simulink model "testF4"  (R2021a)
settings: Solver=FixedStepAuto  StartTime=0.0  StopTime=10.0  RelTol=1e-3  EnableMultiTasking=on
undefined symbols (not defined in the file): ChargingCurrentRequest, DrivingCurrentRqst, OpenCircuitInjection, ShortCircuitInjection, SystemState, SystemState_t
settings Model: Creator=miche  LastModifiedBy=miche
settings OptimizationCC: EnhancedBackFolding=on  PassReuseOutputArgsAs=Individual arguments  ZeroExternalMemoryAtStartup=off  ZeroInternalMemoryAtStartup=off  MaxStackSize=64  OptimizeBlockOrder=speed  DifferentSizesBufferReuse=on  OptimizationCustomize=off  EfficientTunableParamExpr=on
settings DebuggingCC: ParameterTunabilityLossMsg=error  BusObjectLabelMismatch=error
settings HardwareCC: ProdBitPerPointer=32  ProdBitPerSizeT=32  ProdBitPerPtrDiffT=32  ProdLargestAtomicInteger=Long  ProdLargestAtomicFloat=Double  ProdWordSize=32  ProdHWDeviceType=ARM Compatible->ARM Cortex
settings SFSimCC: MATLABDynamicMemAlloc=off
settings RTWCC: SystemTargetFile=ert.tlc  HardwareBoard=STM32F4-Discovery  TemplateMakefile=ert_default_tmf  Toolchain=GNU Tools for ARM Embedded Processors
settings CodeAppCC: ForceParamTrailComments=on  IgnoreCustomStorageClasses=off  OperatorAnnotations=on  SimulinkDataObjDesc=on  SFDataObjDesc=on  InsertBlockDesc=on
settings ERTTargetCC: CodeReplacementLibrary=ARM Cortex-M (Optimized)  ExtModeTransport=1  ExtModeMexFile=ext_serial_win32_comm

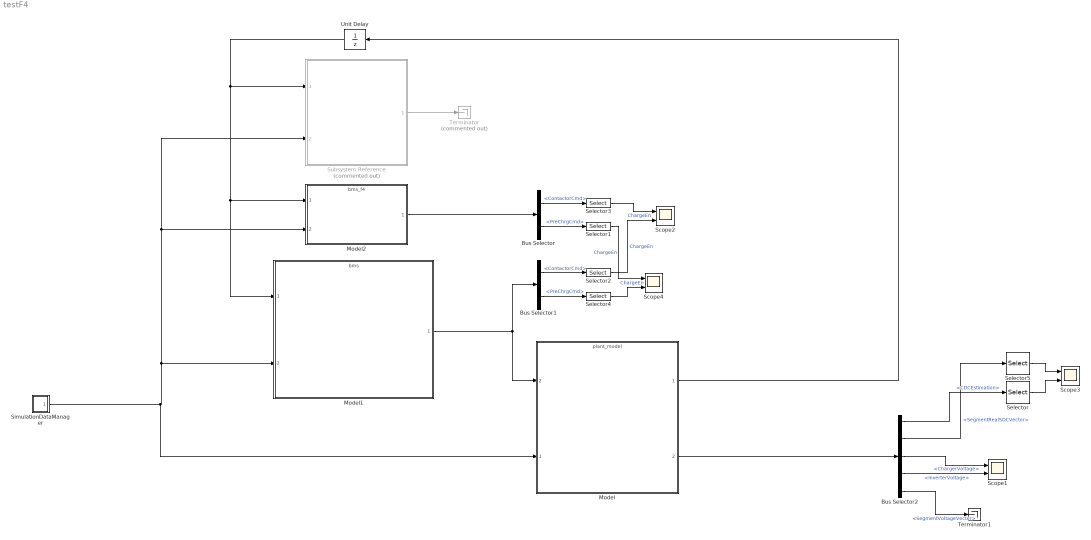
== system testF4 ==
  Bus Selector : BusSelector  OutputSignals=BMSContactorModuleCmd.ContactorCmd,BMSContactorModuleCmd.PreChrgCmd
  Bus Selector1 : BusSelector  OutputSignals=BMSContactorModuleCmd.ContactorCmd,BMSContactorModuleCmd.PreChrgCmd
  Bus Selector2 : BusSelector  OutputSignals=BusSOCEstimation.CDCEstimation,BMSBatteryPackData.SegmentRealSOCVector,SimulationChargerData.ChargerVoltage,SimulationInverterData.InverterVoltage,BMSBatteryPackData.SegmentVoltageVector
  Model : ModelReference  ModelNameDialog=plant_model.slx  SimulationMode=Normal  ModelReferenceVersion=1.26
      settings: PortSchema="{\"entries\":[{\"content\":{\"sides\":[{\"content\":{\"connectorIds\":[\"In2\",\"In1\"]},\"type\":\"ConnectorPlacement.EquallySpacedRectSide\",\"uuid\":\"0f2d7512-e5af-4bec-8093-bd7de674fa12\"},{\"content\":{\"connectorIds\":[\"Out1\",\"Out2\"],\"side\":\"RIGHT\"},\"type\":\"ConnectorPlacement.EquallySpacedRectSide\",\"uuid\":\"ba98a958-4ea7-42df-a4be-bb9f55905ebf\"},{\"content\":{\"connectorIds\":[],\"side\":\"TOP\"},\"type\":\"ConnectorPlacement.EquallySpacedRectSide\",\"uuid\":\"7b43f5d7-e5ff-427f-a248-64d763618be9\"}]},\"type\":\"ConnectorPlacement.EquallySpacedConnector\",\"uuid\":\"924ca3d4-4439-427a-b78a-546ec9901955\"}],\"packageUris\":[\"http://schema.mathworks.com/mf0/Connector/R2020b\"],\"version\":\"1.0\"}"
      mask Display: image('$imagefile'); % Use "Edit Image" on toolstrip to change.
  Model1 : ModelReference  ModelNameDialog=bms.slx  SimulationMode=Normal  ModelReferenceVersion=1.35
      mask Display: image('$imagefile'); % Use "Edit Image" on toolstrip to change.
  Model2 : ModelReference  ModelNameDialog=bms_f4.slx  SimulationMode=Processor-in-the-loop (PIL)  CodeInterface=Top model  ModelReferenceVersion=1.33
  Scope{1..4} (4 alike) : Scope  NumInputPorts=2
  Selector : Selector  NumberOfDimensions=2  InputPortWidth=3  IndexOptions=Index vector (dialog),Index vector (dialog)  Indices=1,1  OutputSizes=1,1
  Selector1 : Selector  InputPortWidth=2  IndexOptions=Index vector (dialog)  Indices=1  OutputSizes=1
  Selector2 : Selector  InputPortWidth=3  IndexOptions=Index vector (dialog)  Indices=1  OutputSizes=1
  Selector3 : Selector  InputPortWidth=3  IndexOptions=Index vector (dialog)  Indices=1  OutputSizes=1
  Selector4 : Selector  InputPortWidth=2  IndexOptions=Index vector (dialog)  Indices=1  OutputSizes=1
  Selector5 : Selector  NumberOfDimensions=2  InputPortWidth=3  IndexOptions=Index vector (dialog),Index vector (dialog)  Indices=1,1  OutputSizes=1,1
  SimulationDataManager : Subsystem
  Subsystem Reference : Subsystem  Commented=on  ReferencedSubsystem=bms_f4_sub
  Terminator : Terminator  Commented=on
  Terminator1 : Terminator
  Unit Delay : UnitDelay  InitialCondition=0.01  SampleTime=-1  HasFrameUpgradeWarning=on
  wires:
  Model/1 -> Unit Delay/1
  Model/2 -> Bus Selector2/1
  Unit Delay/1 -> Model2/1, Model1/1, Subsystem Reference/1
  Model1/1 -> Bus Selector1/1, Model/2
  Subsystem Reference/1 -> Terminator/1
  SimulationDataManager/1(Out1) -> Model/1, Model2/2, Subsystem Reference/2, Model1/2
  Model2/1 -> Bus Selector/1
  Bus Selector/1 -> Selector3/1  "<ContactorCmd>"
  Bus Selector/2 -> Selector1/1  "<PreChrgCmd>"
  Bus Selector1/1 -> Selector2/1  "<ContactorCmd>"
  Bus Selector1/2 -> Selector4/1  "<PreChrgCmd>"
  Selector/1 -> Scope3/2
  Selector5/1 -> Scope3/1
  Bus Selector2/1 -> Selector/1  "<CDCEstimation>"
  Bus Selector2/2 -> Selector5/1  "<SegmentRealSOCVector>"
  Bus Selector2/3 -> Scope1/1  "<ChargerVoltage>"
  Bus Selector2/4 -> Scope1/2  "<InverterVoltage>"
  Bus Selector2/5 -> Terminator1/1  "<SegmentVoltageVector>"
  Selector3/1 -> Scope2/1  "ChargeEn"
  Selector2/1 -> Scope2/2  "ChargeEn"
  Selector1/1 -> Scope4/1  "ChargeEn"
  Selector4/1 -> Scope4/2  "ChargeEn"

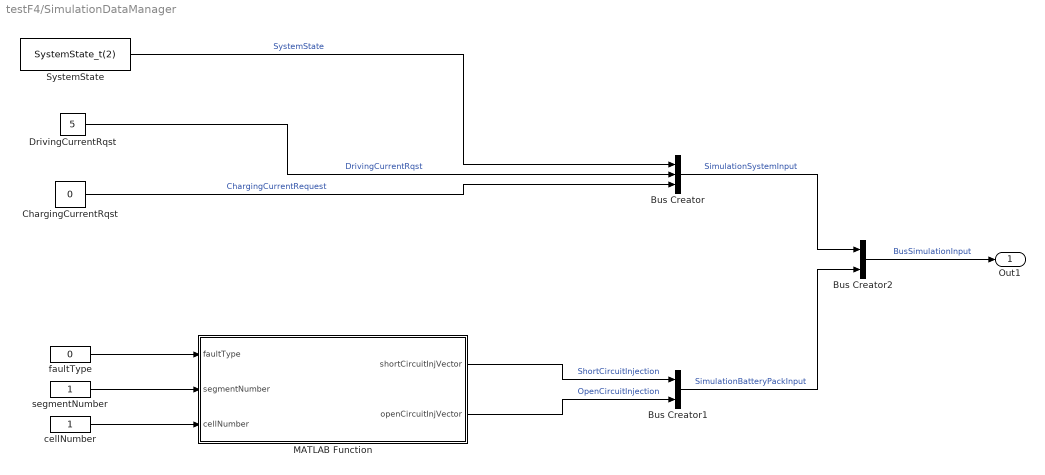
== system testF4/SimulationDataManager ==
  Bus Creator : BusCreator  Inputs=SystemState,DrivingCurrentRqst,ChargingCurrentRequest  OutDataTypeStr=Bus: SimulationSystemInput
  Bus Creator1 : BusCreator  Inputs=ShortCircuitInjection,OpenCircuitInjection  OutDataTypeStr=Bus: SimulationBatteryPackInput
  Bus Creator2 : BusCreator  Inputs=2  OutDataTypeStr=Bus: BusSimulationInput
  ChargingCurrentRqst : Constant  Value=0
  DrivingCurrentRqst : Constant  Value=5
  MATLAB Function : MATLAB Function  TreatAsAtomicUnit=on
  SystemState : Constant  Value=SystemState_t(2)  OutDataTypeStr=Enum: SystemState_t
  cellNumber : Constant
  faultType : Constant  Value=0
  segmentNumber : Constant
  Out1 : Outport
  wires:
  Bus Creator2/1 -> Out1/1  "BusSimulationInput"
  MATLAB Function/2(openCircuitInjVector) -> Bus Creator1/2  "OpenCircuitInjection"
  segmentNumber/1 -> MATLAB Function/2(segmentNumber)
  cellNumber/1 -> MATLAB Function/3(cellNumber)
  MATLAB Function/1(shortCircuitInjVector) -> Bus Creator1/1  "ShortCircuitInjection"
  SystemState/1 -> Bus Creator/1  "SystemState"
  Bus Creator1/1 -> Bus Creator2/2  "SimulationBatteryPackInput"
  faultType/1 -> MATLAB Function/1(faultType)
  ChargingCurrentRqst/1 -> Bus Creator/3  "ChargingCurrentRequest"
  Bus Creator/1 -> Bus Creator2/1  "SimulationSystemInput"
  DrivingCurrentRqst/1 -> Bus Creator/2  "DrivingCurrentRqst"

== matlab function testF4/SimulationDataManager/MATLAB Function ==
  data: faultType input; shortCircuitInjVector output; segmentNumber input; cellNumber input; openCircuitInjVector output
function [shortCircuitInjVector, openCircuitInjVector] = faultInjectionParser(faultType, segmentNumber, cellNumber)

switch(faultType)
    case 0
        shortCircuitInjVector=false(3,10);
        openCircuitInjVector=false(3,10);
    case 1
        shortCircuitInjVector=false(3,10);
        openCircuitInjVector=false(3,10);
        shortCircuitInjVector(segmentNumber, cellNumber)=true;
    case 2
        shortCircuitInjVector=false(3,10);
        openCircuitInjVector=false(3,10);
        openCircuitInjVector(segmentNumber, cellNumber)=true;
    otherwise 
        shortCircuitInjVector=false(3,10);
        openCircuitInjVector=false(3,10);
end
